simulink model "DCmotor"  (R2014b)
settings: Solver=ode45  StartTime=0.0  StopTime=6  RelTol=1e-3
values from neighbouring files (symbols this model uses):
  dv = 1e-5    (= 1e-05)    [DCparamsPD.m]    (also in DCparamsPI.m; DCparamsPID.m)
  eta = 0.74    [DCparamsPD.m]    (also in DCparamsPI.m = 0.75; DCparamsPID.m = 0.75)
  If = s0/r0    [DCparamsPI.m]    (also in DCparamsPID.m)
  imax = 2.5    [DCparamsPD.m]    (also in DCparamsPI.m = 2; DCparamsPID.m = 2; print_control.m = %0.1f;\n',cMode,umax,imax))
  J = 0.05    [DCparamsPD.m]    (also in DCparamsPI.m; DCparamsPID.m; beam_friction.m = 0.000914666666667)
  K = 0.0229    [DCparamsPD.m]    (also in DCparamsPI.m = 0.0214; DCparamsPID.m = 0.0214)
  k_f = [0.072091, 0.040963, -0.003493]    [DCparamsPD.m]    (also in DCparamsPI.m; DCparamsPID.m)
  L = 0.192e-3    (= 0.000192)    [DCparamsPD.m]    (also in DCparamsPI.m = 0.000129; DCparamsPID.m = 0.000129; beam_friction.m = 0.2)
  n = 300564.0/1300.0    (= 231.203076923)    [DCparamsPD.m]    (also in DCparamsPI.m = 149.526172053; DCparamsPID.m = 149.526172053; print_control.m = %0.4f)
  R = 1.83 + 0.33    (= 2.16)    [DCparamsPD.m]    (also in DCparamsPI.m = 1.07; DCparamsPID.m = 1.07; furuta_controller.m = 10; ik_test.m = 0.15925)
  Rc = r0 + s    [DCparamsPD.m]    (also in DCparamsPI.m = s*(r0 + s); DCparamsPID.m = s*(r0 + s))
  Rfc = (s + r0)    [DCparamsPI.m]    (also in DCparamsPID.m = s + r0)
  Sc = s1*s + s0    [DCparamsPD.m]    (also in DCparamsPI.m; DCparamsPID.m = s2*s^2 + s1*s + s0)
  Sfc = sf0 + 0*s    [DCparamsPI.m]    (also in DCparamsPID.m = sf1*s + sf0)
  Tc = t0*(s - w3)    [DCparamsPD.m]    (also in DCparamsPI.m = t0*(s - w3)*(s - w2); DCparamsPID.m = t0*((s-w3)*(s-w4)))
  Tfc = tf1*s + tf0    [DCparamsPI.m]    (also in DCparamsPID.m)
  Ts = 1 / 320    (= 0.003125)    [DCparamsPD.m]    (also in DCparamsPI.m = 0.002; DCparamsPID.m = 0.0016; ik_test.m = 0.0333333333333; read_log_file.m = mean(diff(D{end}.time)))
  umax = 24    [DCparamsPD.m]    (also in DCparamsPI.m; DCparamsPID.m; print_control.m = %0.1f)
libraries: cstblocks x7, simulink x4
settings Model: Creator=vkozma  LastModifiedBy=vkozma
settings DataIOCC: LimitDataPoints=off  SaveTime=off

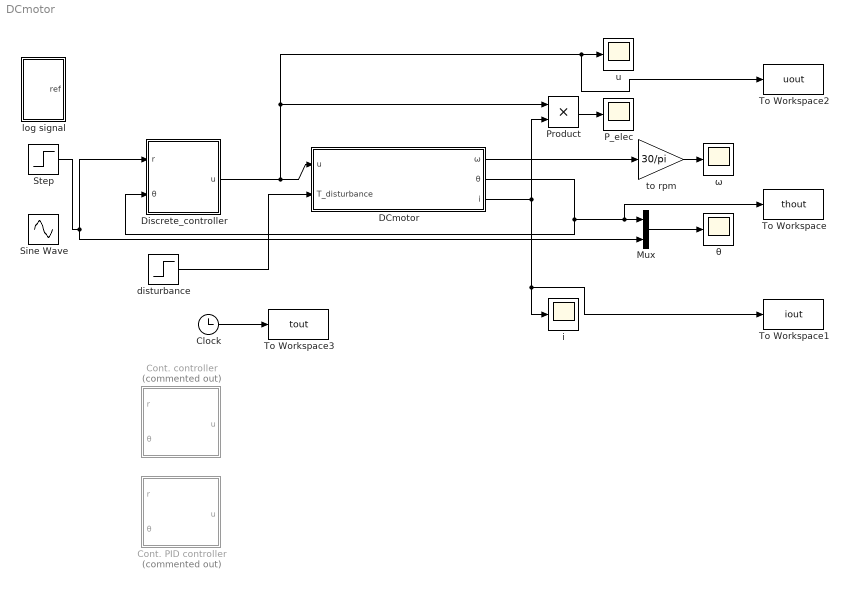
== system DCmotor ==
  Clock : Clock
  Cont. PID controller : Subsystem  Commented=on
  Cont. controller : Subsystem  Commented=on
  DCmotor : Subsystem
  Discrete_controller : Subsystem
  Mux : Mux  Inputs=2
  P_elec : Scope
      settings: SaveName=ScopeData3
  Product : Product
  Sine Wave : Sin  Amplitude=2  Frequency=2*pi  SampleTime=0
  Step : Step  Time=0  After=pi  SampleTime=0
  To Workspace : ToWorkspace  VariableName=thout  SampleTime=1/100
      settings: Save2DSignal=2-D array (concatenate along first dimension)
  To Workspace1 : ToWorkspace  VariableName=iout  SampleTime=1/100
      settings: Save2DSignal=2-D array (concatenate along first dimension)
  To Workspace2 : ToWorkspace  VariableName=uout  SampleTime=1/100
      settings: Save2DSignal=2-D array (concatenate along first dimension)
  To Workspace3 : ToWorkspace  VariableName=tout  SampleTime=1/100
      settings: Save2DSignal=2-D array (concatenate along first dimension)
  disturbance : Step  Time=0  After=0  SampleTime=0
  i : Scope
      settings: SaveName=ScopeData4
  log signal : Subsystem
  to rpm : Gain  Gain=30/pi
  u : Scope
      settings: SaveName=ScopeData2
  θ : Scope
  ω : Scope
  wires:
  DCmotor/2(θ) -> Discrete_controller/2(θ), To Workspace/1, Mux/1
  DCmotor/3(i) -> i/1, To Workspace1/1, Product/2
  Product/1 -> P_elec/1
  Mux/1 -> θ/1
  DCmotor/1(ω) -> to rpm/1
  to rpm/1 -> ω/1
  Step/1 -> Discrete_controller/1(r), Mux/2
  Clock/1 -> To Workspace3/1
  Discrete_controller/1(u) -> To Workspace2/1, u/1, Product/1, DCmotor/1(u)
  disturbance/1 -> DCmotor/2(T_disturbance)

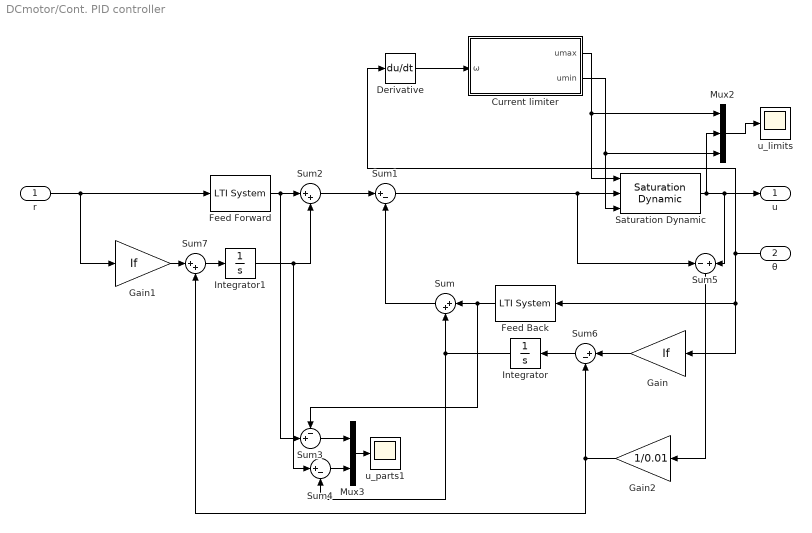
== system DCmotor/Cont. PID controller ==
  r : Inport
  θ : Inport  Port=2
  Current limiter : Subsystem
  Derivative : Derivative
  Feed Back : cstblocks/LTI System  sys=Sfc/Rfc  IC=[]
  Feed Forward : cstblocks/LTI System  sys=Tfc/Rfc  IC=[]
  Gain : Gain  Gain=If
  Gain1 : Gain  Gain=If
  Gain2 : Gain  Gain=1/0.01
  Integrator : Integrator
  Integrator1 : Integrator
  Mux2 : Mux  Inputs=3
  Mux3 : Mux  Inputs=2
  Saturation Dynamic : simulink/Discontinuities/Saturation Dynamic  OutMin=[]  OutMax=[]  OutDataTypeStr=Inherit: Same as second input  OutDataType=fixdt(1, 16)  OutScaling=2^-10  DoSatur=off
  Sum : Sum  Inputs=|++
  Sum1 : Sum  Inputs=|+-
  Sum2 : Sum  Inputs=|++
  Sum3 : Sum  Inputs=-+|
  Sum4 : Sum  Inputs=|+-
  Sum5 : Sum  Inputs=-|+
  Sum6 : Sum  Inputs=|+-
  Sum7 : Sum  Inputs=|++
  u_limits : Scope
      settings: SaveName=ScopeData10
  u_parts1 : Scope
      settings: SaveName=ScopeData13
  u : Outport
  wires:
  r/1 -> Gain1/1, Feed Forward/1
  θ/1 -> Feed Back/1, Gain/1, Derivative/1
  Sum1/1 -> Sum5/1, Saturation Dynamic/2
  Mux2/1 -> u_limits/1
  Current limiter/2(umin) -> Saturation Dynamic/3, Mux2/3
  Current limiter/1(umax) -> Mux2/1, Saturation Dynamic/1
  Saturation Dynamic/1 -> Mux2/2, Sum5/2, u/1
  Derivative/1 -> Current limiter/1(ω)
  Gain/1 -> Sum6/1
  Feed Back/1 -> Sum/1, Sum3/1
  Integrator/1 -> Sum/2, Sum4/2
  Sum/1 -> Sum1/2
  Gain1/1 -> Sum7/1
  Feed Forward/1 -> Sum3/2, Sum2/1
  Integrator1/1 -> Sum2/2, Sum4/1
  Sum2/1 -> Sum1/1
  Mux3/1 -> u_parts1/1
  Sum3/1 -> Mux3/1
  Sum4/1 -> Mux3/2
  Sum6/1 -> Integrator/1
  Sum5/1 -> Gain2/1
  Gain2/1 -> Sum7/2, Sum6/2
  Sum7/1 -> Integrator1/1

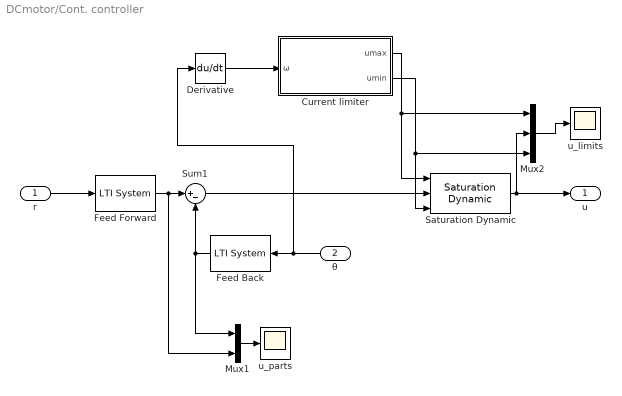
== system DCmotor/Cont. controller ==
  r : Inport
  θ : Inport  Port=2
  Current limiter : Subsystem
  Derivative : Derivative
  Feed Back : cstblocks/LTI System  sys=Sc/Rc  IC=[]
  Feed Forward : cstblocks/LTI System  sys=Tc/Rc  IC=[]
  Mux1 : Mux  Inputs=2
  Mux2 : Mux  Inputs=3
  Saturation Dynamic : simulink/Discontinuities/Saturation Dynamic  OutMin=[]  OutMax=[]  OutDataTypeStr=Inherit: Same as second input  OutDataType=fixdt(1, 16)  OutScaling=2^-10  DoSatur=off
  Sum1 : Sum  Inputs=|+-
  u_limits : Scope
      settings: SaveName=ScopeData10
  u_parts : Scope
      settings: SaveName=ScopeData9
  u : Outport
  wires:
  r/1 -> Feed Forward/1
  θ/1 -> Derivative/1, Feed Back/1
  Mux1/1 -> u_parts/1
  Feed Forward/1 -> Mux1/2, Sum1/1
  Feed Back/1 -> Mux1/1, Sum1/2
  Sum1/1 -> Saturation Dynamic/2
  Mux2/1 -> u_limits/1
  Current limiter/2(umin) -> Saturation Dynamic/3, Mux2/3
  Current limiter/1(umax) -> Mux2/1, Saturation Dynamic/1
  Saturation Dynamic/1 -> Mux2/2, u/1
  Derivative/1 -> Current limiter/1(ω)

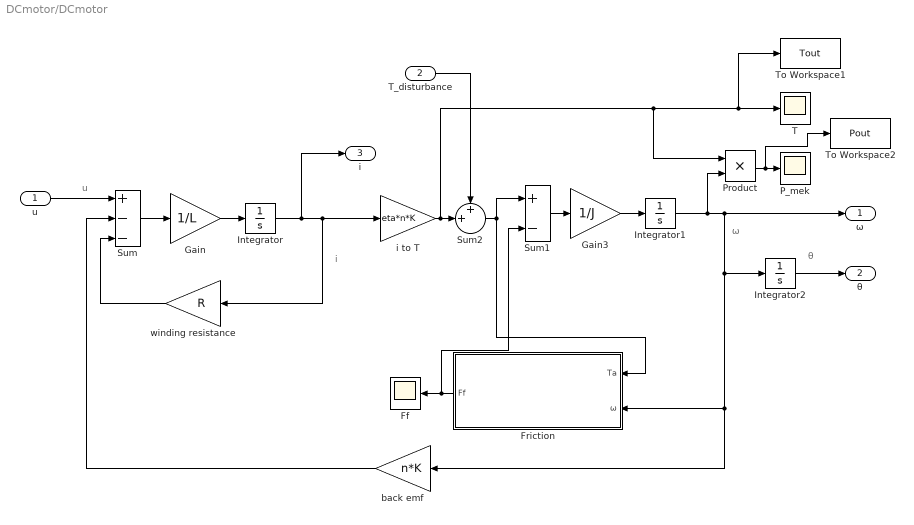
== system DCmotor/DCmotor ==
  note: θ
  note: ω
  note: i
  note: u
  u : Inport
  T_disturbance : Inport  Port=2
  Ff : Scope
      settings: SaveName=ScopeData5
  Friction : Subsystem
  Gain : Gain  Gain=1/L
  Gain3 : Gain  Gain=1/J
  Integrator : Integrator
  Integrator1 : Integrator
  Integrator2 : Integrator
  P_mek : Scope
      settings: SaveName=ScopeData8
  Product : Product
  Sum : Sum  Inputs=+--
  Sum1 : Sum  Inputs=+-
  Sum2 : Sum  Inputs=++|
  T : Scope
      settings: SaveName=ScopeData7
  To Workspace1 : ToWorkspace  VariableName=Tout  SampleTime=1/100
      settings: Save2DSignal=2-D array (concatenate along first dimension)
  To Workspace2 : ToWorkspace  VariableName=Pout  SampleTime=1/100
      settings: Save2DSignal=2-D array (concatenate along first dimension)
  back emf : Gain  Gain=n*K
  i to T : Gain  Gain=eta*n*K
  winding resistance : Gain  Gain=R
  ω : Outport
  θ : Outport  Port=2
  i : Outport  Port=3
  wires:
  u/1 -> Sum/1
  Sum/1 -> Gain/1
  Gain/1 -> Integrator/1
  Integrator/1 -> i/1, winding resistance/1, i to T/1
  winding resistance/1 -> Sum/3
  Sum1/1 -> Gain3/1
  Gain3/1 -> Integrator1/1
  Integrator1/1 -> Product/2, ω/1, Integrator2/1, Friction/2(ω), back emf/1
  i to T/1 -> Sum2/2, Product/1, To Workspace1/1, T/1
  back emf/1 -> Sum/2
  Integrator2/1 -> θ/1
  Product/1 -> To Workspace2/1, P_mek/1
  Friction/1(Ff) -> Sum1/2, Ff/1
  Sum2/1 -> Friction/1(Ta), Sum1/1
  T_disturbance/1 -> Sum2/1

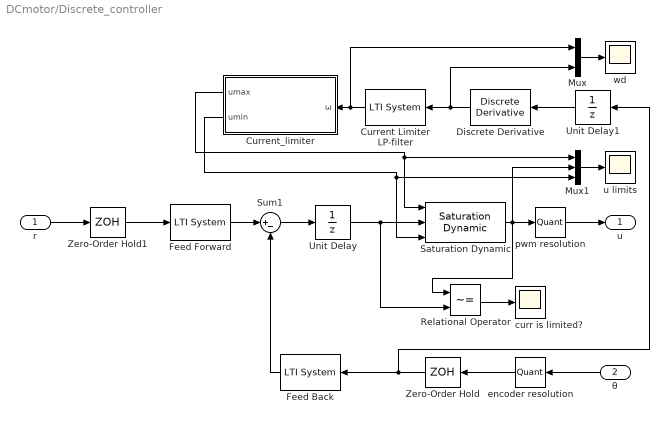
== system DCmotor/Discrete_controller ==
  r : Inport
  θ : Inport  Port=2
  Current Limiter LP-filter : cstblocks/LTI System  sys=Gdcllp  IC=[]
  Current_limiter : Subsystem
  Discrete Derivative : simulink/Discrete/Discrete Derivative  gainval=1.0  ICPrevScaledInput=0.0  InputProcessing=Inherited  OutMin=[]  OutMax=[]  OutDataType=fixdt(1, 16)  OutScaling=2^-10  DoSatur=off
  Feed Back : cstblocks/LTI System  sys=Gdfb  IC=[]
  Feed Forward : cstblocks/LTI System  sys=Gdff  IC=[]
  Mux : Mux  Inputs=2
  Mux1 : Mux  Inputs=3
  Relational Operator : RelationalOperator  Operator=~=  OutDataTypeStr=boolean
  Saturation Dynamic : simulink/Discontinuities/Saturation Dynamic  OutMin=[]  OutMax=[]  OutDataTypeStr=Inherit: Same as second input  OutDataType=fixdt(1, 16)  OutScaling=2^-10  DoSatur=off
  Sum1 : Sum  Inputs=|+-
  Unit Delay : UnitDelay  SampleTime=-1
  Unit Delay1 : UnitDelay  SampleTime=-1
  Zero-Order Hold : ZeroOrderHold  SampleTime=Ts
  Zero-Order Hold1 : ZeroOrderHold  SampleTime=Ts
  curr is limited? : Scope
      settings: SaveName=ScopeData12
  encoder resolution : Quantizer  QuantizationInterval=enc_res
  pwm resolution : Quantizer  QuantizationInterval=volt_res
  u limits : Scope
      settings: SaveName=ScopeData6
  wd : Scope
      settings: SaveName=ScopeData11
  u : Outport
  wires:
  Feed Forward/1 -> Sum1/1
  Feed Back/1 -> Sum1/2
  θ/1 -> encoder resolution/1
  encoder resolution/1 -> Zero-Order Hold/1
  Zero-Order Hold/1 -> Unit Delay1/1, Feed Back/1
  r/1 -> Zero-Order Hold1/1
  Zero-Order Hold1/1 -> Feed Forward/1
  Saturation Dynamic/1 -> pwm resolution/1, Mux1/2, Relational Operator/1
  Sum1/1 -> Unit Delay/1
  Unit Delay/1 -> Relational Operator/2, Saturation Dynamic/2
  Mux/1 -> wd/1
  Mux1/1 -> u limits/1
  Relational Operator/1 -> curr is limited?/1
  Discrete Derivative/1 -> Mux/2, Current Limiter LP-filter/1
  Current_limiter/1(umax) -> Mux1/1, Saturation Dynamic/1
  Current_limiter/2(umin) -> Saturation Dynamic/3, Mux1/3
  Current Limiter LP-filter/1 -> Mux/1, Current_limiter/1(ω)
  pwm resolution/1 -> u/1
  Unit Delay1/1 -> Discrete Derivative/1

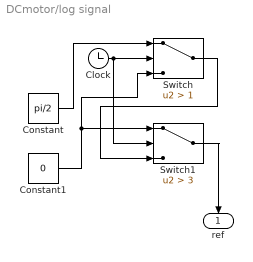
== system DCmotor/log signal ==
  Clock : Clock
  Constant : Constant  Value=pi/2
  Constant1 : Constant  Value=0
  Switch : Switch  Criteria=u2 > Threshold  Threshold=1
  Switch1 : Switch  Criteria=u2 > Threshold  Threshold=3
  ref : Outport
  wires:
  Constant1/1 -> Switch1/1, Switch/3
  Clock/1 -> Switch1/2, Switch/2
  Constant/1 -> Switch/1
  Switch1/1 -> ref/1
  Switch/1 -> Switch1/3

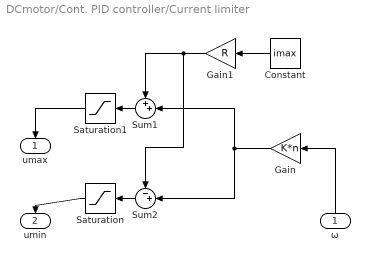
== system DCmotor/Cont. PID controller/Current limiter ==
  ω : Inport
  Constant : Constant  Value=imax
  Gain : Gain  Gain=K*n
  Gain1 : Gain  Gain=R
  Saturation : Saturate  UpperLimit=umax  LowerLimit=-umax
  Saturation1 : Saturate  UpperLimit=umax  LowerLimit=-umax
  Sum1 : Sum  Inputs=++|
  Sum2 : Sum  Inputs=-+|
  umax : Outport
  umin : Outport  Port=2
  wires:
  Sum2/1 -> Saturation/1
  ω/1 -> Gain/1
  Gain/1 -> Sum2/2, Sum1/2
  Constant/1 -> Gain1/1
  Gain1/1 -> Sum2/1, Sum1/1
  Sum1/1 -> Saturation1/1
  Saturation/1 -> umin/1
  Saturation1/1 -> umax/1

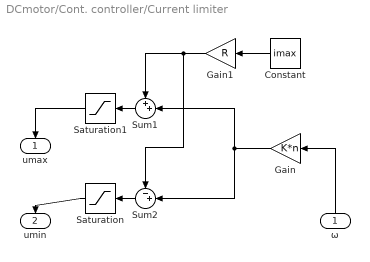
== system DCmotor/Cont. controller/Current limiter ==
  ω : Inport
  Constant : Constant  Value=imax
  Gain : Gain  Gain=K*n
  Gain1 : Gain  Gain=R
  Saturation : Saturate  UpperLimit=umax  LowerLimit=-umax
  Saturation1 : Saturate  UpperLimit=umax  LowerLimit=-umax
  Sum1 : Sum  Inputs=++|
  Sum2 : Sum  Inputs=-+|
  umax : Outport
  umin : Outport  Port=2
  wires:
  Sum2/1 -> Saturation/1
  ω/1 -> Gain/1
  Gain/1 -> Sum2/2, Sum1/2
  Constant/1 -> Gain1/1
  Gain1/1 -> Sum2/1, Sum1/1
  Sum1/1 -> Saturation1/1
  Saturation/1 -> umin/1
  Saturation1/1 -> umax/1

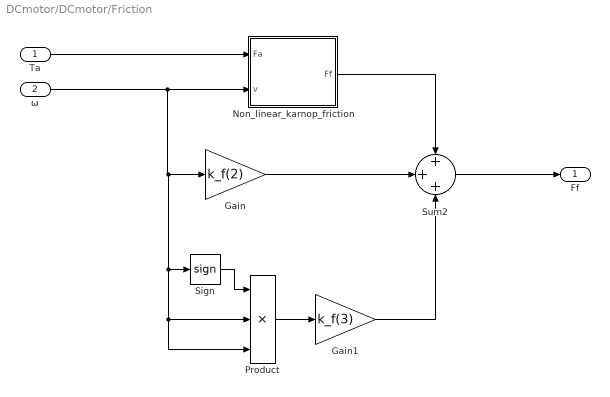
== system DCmotor/DCmotor/Friction ==
  Ta : Inport
  ω : Inport  Port=2
  Gain : Gain  Gain=k_f(2)
  Gain1 : Gain  Gain=k_f(3)
  Non_linear_karnop_friction : Subsystem
  Product : Product  Inputs=3
  Sign : Signum
  Sum2 : Sum  Inputs=+++
  Ff : Outport
  wires:
  ω/1 -> Product/3, Product/2, Sign/1, Gain/1, Non_linear_karnop_friction/2(v)
  Ta/1 -> Non_linear_karnop_friction/1(Fa)
  Sum2/1 -> Ff/1
  Non_linear_karnop_friction/1(Ff) -> Sum2/1
  Gain/1 -> Sum2/2
  Sign/1 -> Product/1
  Product/1 -> Gain1/1
  Gain1/1 -> Sum2/3

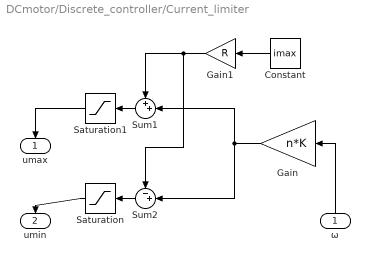
== system DCmotor/Discrete_controller/Current_limiter ==
  ω : Inport
  Constant : Constant  Value=imax
  Gain : Gain  Gain=n*K
  Gain1 : Gain  Gain=R
  Saturation : Saturate  UpperLimit=umax  LowerLimit=-umax
  Saturation1 : Saturate  UpperLimit=umax  LowerLimit=-umax
  Sum1 : Sum  Inputs=++|
  Sum2 : Sum  Inputs=-+|
  umax : Outport
  umin : Outport  Port=2
  wires:
  Sum2/1 -> Saturation/1
  ω/1 -> Gain/1
  Gain/1 -> Sum2/2, Sum1/2
  Constant/1 -> Gain1/1
  Gain1/1 -> Sum2/1, Sum1/1
  Sum1/1 -> Saturation1/1
  Saturation/1 -> umin/1
  Saturation1/1 -> umax/1

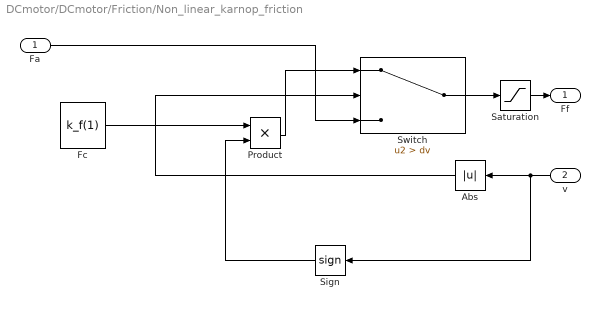
== system DCmotor/DCmotor/Friction/Non_linear_karnop_friction ==
  Fa : Inport
  v : Inport  Port=2
  Abs : Abs
  Fc : Constant  Value=k_f(1)
  Product : Product  RndMeth=Zero
  Saturation : Saturate  UpperLimit=k_f(1)  LowerLimit=-k_f(1)
  Sign : Signum
  Switch : Switch  Criteria=u2 > Threshold  Threshold=dv
  Ff : Outport
  wires:
  Sign/1 -> Product/2
  Fc/1 -> Product/1
  Abs/1 -> Switch/2
  Fa/1 -> Switch/3
  v/1 -> Abs/1, Sign/1
  Switch/1 -> Saturation/1
  Saturation/1 -> Ff/1
  Product/1 -> Switch/1
